simulink model "reduced_model_PT1_J3"  (R2019b)
settings: Solver=ode1  StartTime=0.0  StopTime=2.4  FixedStep=0.001  RelTol=1e-3
undefined symbols (not defined in the file): __PRM__SERIALIZED__DATA__, jointVelocityLowerLimit, jointVelocityUpperLimit, SubsystemReferenceBlock
libraries: simulink x1, robotmaniplib x1
settings Model: Creator=Robot  LastModifiedBy=Robot

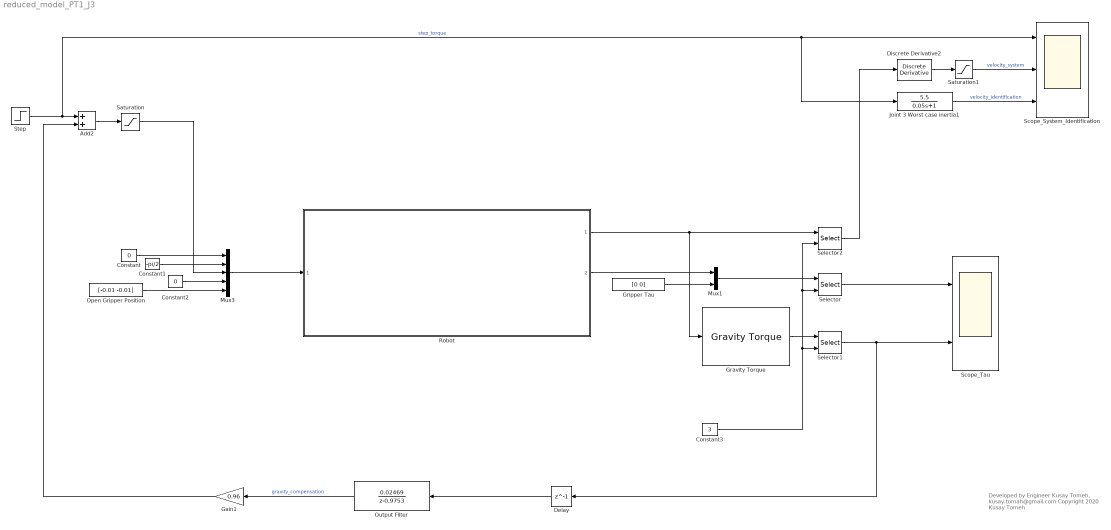
== system reduced_model_PT1_J3 ==
  note: Developed by Engineer Kusay Tomeh,
      | kusay.tomah@gmail.com
      | Copyright 2020 Kusay Tomeh
  " Gripper Tau" : Constant  Value=[0 0]
  Add2 : Sum
  Constant : Constant  Value=0
  Constant1 : Constant  Value=-pi/2
  Constant2 : Constant  Value=0
  Constant3 : Constant  Value=3
  Delay : Delay  DelayLength=1
  Discrete Derivative2 : simulink/Discrete/Discrete Derivative  gainval=1  ICPrevScaledInput=0.0  OutMin=[]  OutMax=[]  OutDataType=fixdt(1, 16)  OutScaling=2^-10  DoSatur=off
  Gain1 : Gain  Gain=0.96
  Gravity Torque : robotmaniplib/Gravity Torque  RigidBodyTree=robot  SimulateUsing=Interpreted execution
      settings: SourceProductName=Robotics System Toolbox
  Joint 3 Worst case inertia1 : TransferFcn  Numerator=[5.5]  Denominator=[0.05 1]
  Mux1 : Mux  Inputs=2
  Mux3 : Mux  Inputs=5
  Open Gripper Position : Constant  Value=[-0.01 -0.01]
  Output Filter : DiscreteTransferFcn  Numerator=0.02469  Denominator=[1 -0.9753]
  Robot : Subsystem  BlockKeywords=__PRM__SERIALIZED__DATA__:SubsystemReferenceBlock  ReferencedSubsystem=RobotModelWithFloor
  Saturation : Saturate  UpperLimit=2  LowerLimit=-2
  Saturation1 : Saturate  UpperLimit=jointVelocityUpperLimit  LowerLimit=jointVelocityLowerLimit
  Scope_System_Identification : Scope  NumInputPorts=3
  Scope_Tau : Scope  NumInputPorts=2
  Selector : Selector  InputPortWidth=6  IndexOptions=Index vector (port)  Indices=[1 3]  OutputSizes=1
  Selector1 : Selector  InputPortWidth=6  IndexOptions=Index vector (port)  Indices=[1 3]  OutputSizes=1
  Selector2 : Selector  InputPortWidth=6  IndexOptions=Index vector (port)  Indices=[1 3]  OutputSizes=1
  Step : Step  Time=2
  wires:
  Gravity Torque/1 -> Selector1/1
  Discrete Derivative2/1 -> Saturation1/1
  Constant3/1 -> Selector2/2, Selector/2, Selector1/2
  Constant2/1 -> Mux3/4
  Robot/1 -> Gravity Torque/1, Selector2/1
  Open Gripper Position/1 -> Mux3/5
  Constant/1 -> Mux3/1
  Selector2/1 -> Discrete Derivative2/1
  Add2/1 -> Saturation/1
  Mux3/1 -> Robot/1
  Selector/1 -> Scope_Tau/1
  " Gripper Tau"/1 -> Mux1/2
  Robot/2 -> Mux1/1
  Mux1/1 -> Selector/1
  Step/1 -> Joint 3 Worst case inertia1/1, Scope_System_Identification/1, Add2/1  "step_torque"
  Selector1/1 -> Delay/1, Scope_Tau/2
  Output Filter/1 -> Gain1/1  "gravity_compensation"
  Gain1/1 -> Add2/2
  Delay/1 -> Output Filter/1
  Saturation1/1 -> Scope_System_Identification/2  "velocity_system"
  Constant1/1 -> Mux3/2
  Saturation/1 -> Mux3/3
  Joint 3 Worst case inertia1/1 -> Scope_System_Identification/3  "velocity_identification"
